simulink model "real_time_5"  (R2024b)
settings: Solver=ode5  StartTime=0.0  StopTime=5  FixedStep=0.001  RelTol=1e-3
values from neighbouring files (symbols this model uses):
  A0 = A22_prime-L*A12_prime    [code_ali.m]    (also in lab2_challenge_ali.m)
  B0 = [B_prime(2)-L*B_prime(1),A0*L+A_prime(2,1)-L*A_prime(1,1)]    [code_ali.m]    (also in lab2_challenge_ali.m)
  C0 = T_trsf*[0;1]    [code_ali.m]    (also in lab2_challenge_ali.m)
  D0 = T_trsf*[0,1;0,L]    [code_ali.m]    (also in lab2_challenge_ali.m)
  degs2rpm = 60/360    (= 0.166666666667)    [Init_ali.m]
  K2 = K_robust(2:3)    [code_ali.m]    (also in lab2_challenge_ali.m)
  KI = K_robust(1)    [code_ali.m]    (also in lab2_challenge_ali.m)
  Nu = Ans(3,1)    [code_ali.m]    (also in lab2_challenge_ali.m)
  Nx = Ans(1:2,1)    [code_ali.m]    (also in lab2_challenge_ali.m)
  rpm2rads = 2*pi/60    (= 0.10471975512)    [Init_ali.m]
undefined symbols (not defined in the file or in its folder): National_Instruments, PCI
libraries: sldrtlib x3
settings Model: SimulationMode=external  ExtModeTrigDuration=1000001  Creator=galeazzolu  LastModifiedBy=Ali
settings DataIOCC: ReturnWorkspaceOutputs=off
settings HardwareCC: ProdBitPerLong=64  ProdHWDeviceType=Intel->x86-64 (Linux 64)
settings RTWCC: Description=Simulink Desktop Real-Time  SystemTargetFile=sldrt.tlc  TemplateMakefile=sldrt.tmf  RTWCompilerOptimization=on
settings CodeAppCC: MaxIdLength=95
settings SimulinkDesktopRealTimeCC: TargetLibSuffix=_sldrt.a  TargetPreCompLibLocation=C:\Program Files\MATLAB\R2024b\toolbox\sldrt\lib\win64  ParMdlRefBuildCompliant=on

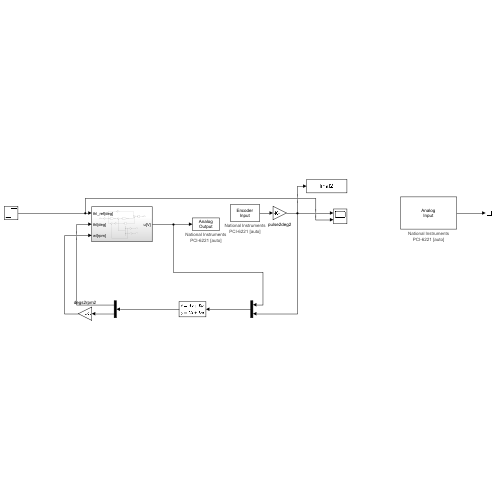
[thumbnail: Simulink's stored preview of the top-level diagram]
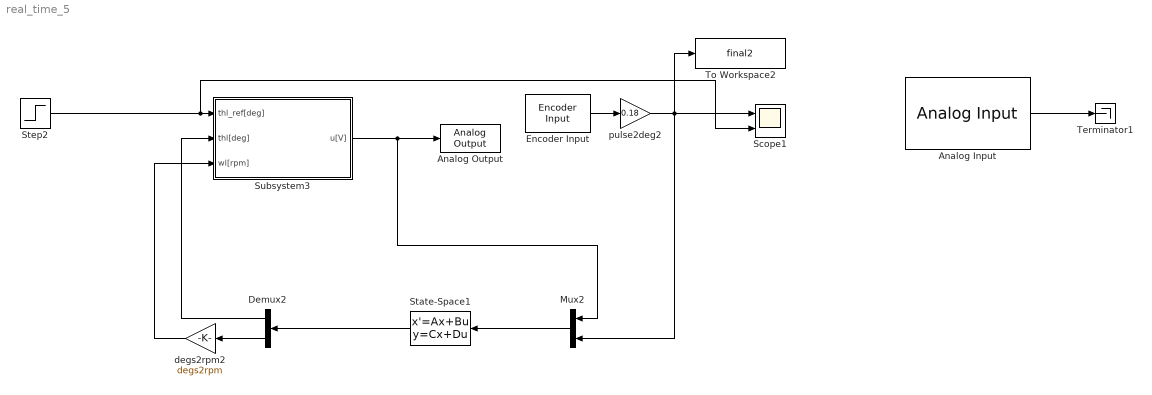
== system real_time_5 ==
  Analog Input : sldrtlib/Analog Input  SampleTime=-1  MaxMissedTicks=10  ShowMissedTicks=off  YieldWhenWaiting=off  DrvName=National_Instruments/PCI-6221  DrvAddress=4294967295  DrvOptions=[0 0 0 2 0]  Channels=[1,2]  RangeMode=1  VoltRange=1  DataType=1
      settings: AttributesFormatString=National Instruments\nPCI-6221 [auto]
  Analog Output : sldrtlib/Analog Output  SampleTime=-1  MaxMissedTicks=10  ShowMissedTicks=off  YieldWhenWaiting=off  DrvName=National_Instruments/PCI-6221  DrvAddress=4294967295  DrvOptions=[0 0 0 2 0]  Channels=1  RangeMode=1  VoltRange=1  InitialValue=0  FinalValue=0
      settings: AttributesFormatString=National Instruments\nPCI-6221 [auto]
  Demux2 : Demux  Outputs=2
  Encoder Input : sldrtlib/Encoder Input  SampleTime=-1  MaxMissedTicks=10  ShowMissedTicks=off  YieldWhenWaiting=off  DrvName=National_Instruments/PCI-6221  DrvAddress=4294967295  DrvOptions=[0 0 0 2 0]  Channels=1  QuadMode=3  IndexPulse=1  InputFilter=Inf  DataType=1
      settings: AttributesFormatString=National Instruments\nPCI-6221 [auto]
  Mux2 : Mux  Inputs=2
  Scope1 : Scope  NumInputPorts=2
  State-Space1 : StateSpace  A=A0  B=B0  C=C0  D=D0  InitialCondition=0
  Step2 : Step  Time=0  After=40  SampleTime=0
  Subsystem3 : Subsystem
  Terminator1 : Terminator
  To Workspace2 : ToWorkspace  VariableName=final2  SaveFormat=Structure With Time  SampleTime=-1
  degs2rpm2 : Gain  Gain=degs2rpm
  pulse2deg2 : Gain  Gain=0.18
  wires:
  Analog Input/1 -> Terminator1/1
  Subsystem3/1(u[V]) -> Analog Output/1, Mux2/1
  pulse2deg2/1 -> To Workspace2/1, Scope1/1, Mux2/2
  Mux2/1 -> State-Space1/1
  degs2rpm2/1 -> Subsystem3/3(wl[rpm])
  Step2/1 -> Scope1/2, Subsystem3/1(thl_ref[deg])
  Demux2/1 -> Subsystem3/2(thl[deg])
  Demux2/2 -> degs2rpm2/1
  Encoder Input/1 -> pulse2deg2/1
  State-Space1/1 -> Demux2/1

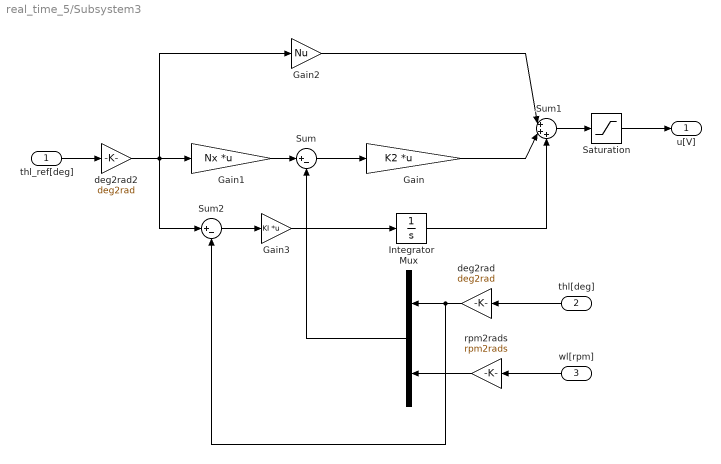
== system real_time_5/Subsystem3 ==
  thl_ref[deg] : Inport
  thl[deg] : Inport  Port=2
  wl[rpm] : Inport  Port=3
  Gain : Gain  Gain=K2  Multiplication=Matrix(K*u)
  Gain1 : Gain  Gain=Nx  Multiplication=Matrix(K*u)
  Gain2 : Gain  Gain=Nu
  Gain3 : Gain  Gain=KI  Multiplication=Matrix(K*u)
  Integrator : Integrator
  Mux : Mux  Inputs=2
  Saturation : Saturate  UpperLimit=12  LowerLimit=-12
  Sum : Sum  Inputs=|+-
  Sum1 : Sum  Inputs=|+++
  Sum2 : Sum  Inputs=|+-
  deg2rad : Gain  Gain=deg2rad
  deg2rad2 : Gain  Gain=deg2rad
  rpm2rads : Gain  Gain=rpm2rads
  u[V] : Outport
  wires:
  thl[deg]/1 -> deg2rad/1
  wl[rpm]/1 -> rpm2rads/1
  deg2rad/1 -> Mux/1, Sum2/2
  rpm2rads/1 -> Mux/2
  Sum/1 -> Gain/1
  Gain1/1 -> Sum/1
  thl_ref[deg]/1 -> deg2rad2/1
  deg2rad2/1 -> Gain1/1, Sum2/1, Gain2/1
  Gain2/1 -> Sum1/1
  Gain/1 -> Sum1/2
  Sum1/1 -> Saturation/1
  Saturation/1 -> u[V]/1
  Integrator/1 -> Sum1/3
  Sum2/1 -> Gain3/1
  Gain3/1 -> Integrator/1
  Mux/1 -> Sum/2
